simulink model "LinearSolver_System"  (R2021a)
settings: Solver=VariableStepAuto  StartTime=0.0  StopTime=1000  RelTol=1e-3
undefined symbols (not defined in the file or in its folder): AXI4, Lite
libraries: hdlBasic x415, xbsIndex_r4 x1
(part 1 of 4)
settings Model: Creator=hl116  LastModifiedBy=user

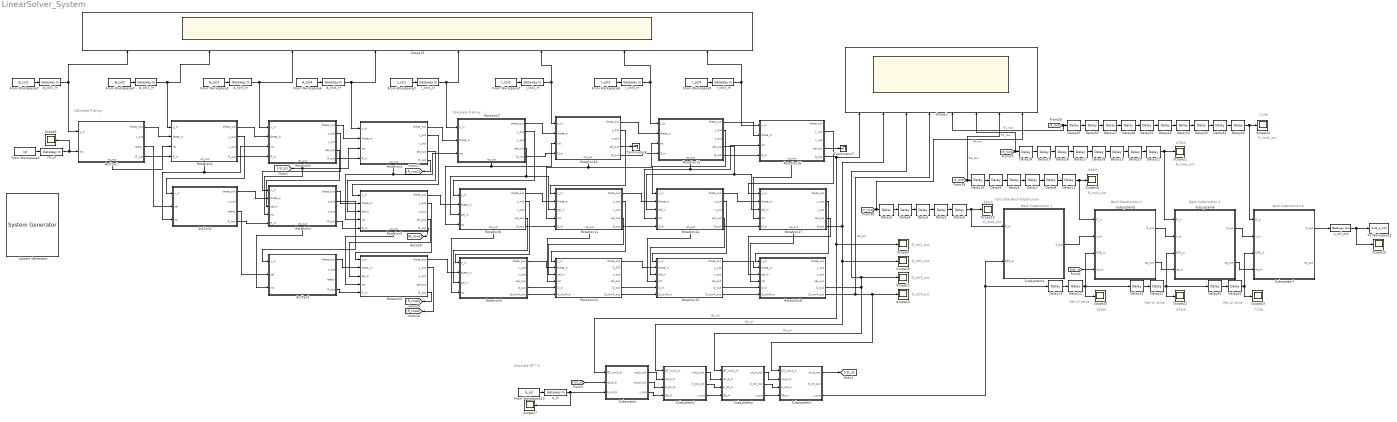
== system LinearSolver_System ==
  note: Q_col2_out
  note: 717th
  note: R_row1_out
  note: R_row3_out
  note: Q_col3_out
  note: Calculate QT * b
  note: 675th
  note: Calculate R Array
  note: y_out
  note: 717th
  note: Back Substitution 2
  note: Get y3 value
  note: Q_col1_out
  note: 633th
  note: 591th
  note: Calculate Q Array
  note: Back Substitution 4
  note: Back Substitution 1
  note: 675th
  note: Q_col4_out
  note: Get y2 value
  note: R_row2_out
  note: R_row4_out
  note: Get y2 value
  note: Calculate Back Substitution
  note: Back Substitution 3
  note: 633th
  " System Generator" : xbsIndex_r4/ System Generator  Tag=genX  xilinxfamily=zynq  part=xc7z020  speed=-1  package=clg484  synthesis_tool=Vivado  clock_wrapper=Clock Enables  directory=./netlist_project6_final  proj_type=Vivado  Synth_file=Vivado Synthesis Defaults  Impl_file=Vivado Implementation Defaults  testbench=off  simulink_period=1  sysclk_period=10  dcm_input_clock_period=10  incr_netlist=off  trim_vbits=Everywhere in SubSystem  dbl_ovrd=According to Block Masks  core_generation=According to Block Masks  run_coregen=off  deprecated_control=off  eval_field=0  block_type=sysgen
  A_col1_In : hdlBasic/Gateway In  gui_display_data_type=Fixed-point  arith_type=Signed (2's comp)  n_bits=16  bin_pt=13  preci_type=Single  exp_width=8  frac_width=24  rows=1  columns=1  quantization="Round  (unbiased: +/- Inf)"  overflow=Saturate  period=1  UseAsADC=off  ADCChannel='1'  interface=AXI4-Lite  automatic_assignment=on  address_offset=hex2dec('00')  intf_name=''  intf_description=''  default_value=0  timing_constraint=None  locs_specified=off  LOCs={}  io_standard={}  inherit_from_input=off  hdl_port=on  XmcBlockStatus=1  maskContainerNames=group4  block_type=gatewayin  block_config=sysgen:gateway_in_config  block_width_w=590  block_height_w=620  block_width=640  block_height=850
  A_col2_In : hdlBasic/Gateway In  gui_display_data_type=Fixed-point  arith_type=Signed (2's comp)  n_bits=16  bin_pt=13  preci_type=Single  exp_width=8  frac_width=24  rows=1  columns=1  quantization="Round  (unbiased: +/- Inf)"  overflow=Saturate  period=1  UseAsADC=off  ADCChannel='1'  interface=AXI4-Lite  automatic_assignment=on  address_offset=hex2dec('00')  intf_name=''  intf_description=''  default_value=0  timing_constraint=None  locs_specified=off  LOCs={}  io_standard={}  inherit_from_input=off  hdl_port=on  XmcBlockStatus=1  maskContainerNames=group4  block_type=gatewayin  block_config=sysgen:gateway_in_config  block_width_w=590  block_height_w=620  block_width=640  block_height=850
  A_col3_In : hdlBasic/Gateway In  gui_display_data_type=Fixed-point  arith_type=Signed (2's comp)  n_bits=16  bin_pt=13  preci_type=Single  exp_width=8  frac_width=24  rows=1  columns=1  quantization="Round  (unbiased: +/- Inf)"  overflow=Saturate  period=1  UseAsADC=off  ADCChannel='1'  interface=AXI4-Lite  automatic_assignment=on  address_offset=hex2dec('00')  intf_name=''  intf_description=''  default_value=0  timing_constraint=None  locs_specified=off  LOCs={}  io_standard={}  inherit_from_input=off  hdl_port=on  XmcBlockStatus=1  maskContainerNames=group4  block_type=gatewayin  block_config=sysgen:gateway_in_config  block_width_w=590  block_height_w=620  block_width=640  block_height=850
  A_col4_In : hdlBasic/Gateway In  gui_display_data_type=Fixed-point  arith_type=Signed (2's comp)  n_bits=16  bin_pt=13  preci_type=Single  exp_width=8  frac_width=24  rows=1  columns=1  quantization="Round  (unbiased: +/- Inf)"  overflow=Saturate  period=1  UseAsADC=off  ADCChannel='1'  interface=AXI4-Lite  automatic_assignment=on  address_offset=hex2dec('00')  intf_name=''  intf_description=''  default_value=0  timing_constraint=None  locs_specified=off  LOCs={}  io_standard={}  inherit_from_input=off  hdl_port=on  XmcBlockStatus=1  maskContainerNames=group4  block_type=gatewayin  block_config=sysgen:gateway_in_config  block_width_w=590  block_height_w=620  block_width=640  block_height=850
  ArcTan1 : Subsystem
      settings: PortSchema="{\"entries\":[{\"content\":{\"sides\":[{\"content\":{\"connectorIds\":[\"In1\",\"In2\"]},\"type\":\"ConnectorPlacement.EquallySpacedRectSide\",\"uuid\":\"caf108fa-2686-498d-a22a-9c5b9b2bbc42\"},{\"content\":{\"connectorIds\":[\"Out1\",\"Out2\",\"Out3\",\"Out4\"],\"side\":\"RIGHT\"},\"type\":\"ConnectorPlacement.EquallySpacedRectSide\",\"uuid\":\"907814ff-b94e-448a-ba79-154ff3b88489\"},{\"content\":{\"connectorIds\":[],\"side\":\"TOP\"},\"type\":\"ConnectorPlacement.EquallySpacedRectSide\",\"uuid\":\"95b6304b-e160-4f42-b0ad-ca1595d39137\"},{\"content\":{\"connectorIds\":[\"Out5\"],\"side\":\"BOTTOM\"},\"type\":\"ConnectorPlacement.EquallySpacedRectSide\",\"uuid\":\"89d2f461-a37a-483a-b43d-da0d10659910\"}]},\"type\":\"ConnectorPlacement.EquallySpacedConnector\",\"uuid\":\"3f5841f0-ef35-46d4-afb7-d5d76fae65b0\"}],\"packageUris\":[\"http://schema.mathworks.com/mf0/Connector/R2020b\"],\"version\":\"1.0\"}"
  ArcTan2 : Subsystem
  ArcTan3 : Subsystem
  Delay{1..35} (35 alike) : hdlBasic/Delay  rst=off  en=off  latency=42  reg_retiming=off  XmcBlockStatus=1  maskContainerNames=group1  block_type=delay  block_config=sysgen:Delay_config
  From Workspace1 : FromWorkspace  VariableName=I_col1
  From Workspace10 : FromWorkspace  VariableName=b_col
  From Workspace2 : FromWorkspace  VariableName=rst
  From Workspace3 : FromWorkspace  VariableName=A_col1
  From Workspace4 : FromWorkspace  VariableName=A_col2
  From Workspace5 : FromWorkspace  VariableName=A_col3
  From Workspace6 : FromWorkspace  VariableName=A_col4
  From Workspace7 : FromWorkspace  VariableName=I_col2
  From Workspace8 : FromWorkspace  VariableName=I_col3
  From Workspace9 : FromWorkspace  VariableName=I_col4
  I_col1_In : hdlBasic/Gateway In  gui_display_data_type=Fixed-point  arith_type=Signed (2's comp)  n_bits=16  bin_pt=13  preci_type=Single  exp_width=8  frac_width=24  rows=1  columns=1  quantization="Round  (unbiased: +/- Inf)"  overflow=Saturate  period=1  UseAsADC=off  ADCChannel='1'  interface=AXI4-Lite  automatic_assignment=on  address_offset=hex2dec('00')  intf_name=''  intf_description=''  default_value=0  timing_constraint=None  locs_specified=off  LOCs={}  io_standard={}  inherit_from_input=off  hdl_port=on  XmcBlockStatus=1  maskContainerNames=group4  block_type=gatewayin  block_config=sysgen:gateway_in_config  block_width_w=590  block_height_w=620  block_width=640  block_height=850
  I_col2_In : hdlBasic/Gateway In  gui_display_data_type=Fixed-point  arith_type=Signed (2's comp)  n_bits=16  bin_pt=13  preci_type=Single  exp_width=8  frac_width=24  rows=1  columns=1  quantization="Round  (unbiased: +/- Inf)"  overflow=Saturate  period=1  UseAsADC=off  ADCChannel='1'  interface=AXI4-Lite  automatic_assignment=on  address_offset=hex2dec('00')  intf_name=''  intf_description=''  default_value=0  timing_constraint=None  locs_specified=off  LOCs={}  io_standard={}  inherit_from_input=off  hdl_port=on  XmcBlockStatus=1  maskContainerNames=group4  block_type=gatewayin  block_config=sysgen:gateway_in_config  block_width_w=590  block_height_w=620  block_width=640  block_height=850
  I_col3_In : hdlBasic/Gateway In  gui_display_data_type=Fixed-point  arith_type=Signed (2's comp)  n_bits=16  bin_pt=13  preci_type=Single  exp_width=8  frac_width=24  rows=1  columns=1  quantization="Round  (unbiased: +/- Inf)"  overflow=Saturate  period=1  UseAsADC=off  ADCChannel='1'  interface=AXI4-Lite  automatic_assignment=on  address_offset=hex2dec('00')  intf_name=''  intf_description=''  default_value=0  timing_constraint=None  locs_specified=off  LOCs={}  io_standard={}  inherit_from_input=off  hdl_port=on  XmcBlockStatus=1  maskContainerNames=group4  block_type=gatewayin  block_config=sysgen:gateway_in_config  block_width_w=590  block_height_w=620  block_width=640  block_height=850
  I_col4_In : hdlBasic/Gateway In  gui_display_data_type=Fixed-point  arith_type=Signed (2's comp)  n_bits=16  bin_pt=13  preci_type=Single  exp_width=8  frac_width=24  rows=1  columns=1  quantization="Round  (unbiased: +/- Inf)"  overflow=Saturate  period=1  UseAsADC=off  ADCChannel='1'  interface=AXI4-Lite  automatic_assignment=on  address_offset=hex2dec('00')  intf_name=''  intf_description=''  default_value=0  timing_constraint=None  locs_specified=off  LOCs={}  io_standard={}  inherit_from_input=off  hdl_port=on  XmcBlockStatus=1  maskContainerNames=group4  block_type=gatewayin  block_config=sysgen:gateway_in_config  block_width_w=590  block_height_w=620  block_width=640  block_height=850
  Rotation1 : Subsystem
      settings: PortSchema="{\"entries\":[{\"content\":{\"sides\":[{\"content\":{\"connectorIds\":[\"In1\",\"In2\",\"In3\",\"In4\"]},\"type\":\"ConnectorPlacement.EquallySpacedRectSide\",\"uuid\":\"c3e45f34-1196-45a4-bcee-69f3d7240640\"},{\"content\":{\"connectorIds\":[\"Out1\",\"Out2\",\"Out3\",\"Out4\"],\"side\":\"RIGHT\"},\"type\":\"ConnectorPlacement.EquallySpacedRectSide\",\"uuid\":\"79e1b465-033e-4299-96e2-1b0cd35cf0c2\"},{\"content\":{\"connectorIds\":[],\"side\":\"TOP\"},\"type\":\"ConnectorPlacement.EquallySpacedRectSide\",\"uuid\":\"795b3f8d-3c8d-4387-9426-6b007387498d\"},{\"content\":{\"connectorIds\":[\"Out5\"],\"side\":\"BOTTOM\"},\"type\":\"ConnectorPlacement.EquallySpacedRectSide\",\"uuid\":\"45ba46a5-4748-4846-a91b-1f19bc6fdcdf\"}]},\"type\":\"ConnectorPlacement.EquallySpacedConnector\",\"uuid\":\"22f19e15-548a-4ba4-8f17-e0c3567ab6b5\"}],\"packageUris\":[\"http://schema.mathworks.com/mf0/Connector/R2020b\"],\"version\":\"1.0\"}"
  Rotation10 : Subsystem
      settings: PortSchema="{\"entries\":[{\"content\":{\"sides\":[{\"content\":{\"connectorIds\":[\"In1\",\"In2\",\"In3\",\"In4\"]},\"type\":\"ConnectorPlacement.EquallySpacedRectSide\",\"uuid\":\"068d33f8-cdb2-46c3-8301-e7e31b8e2d88\"},{\"content\":{\"connectorIds\":[\"Out1\",\"Out2\",\"Out3\",\"Out4\",\"Out5\"],\"side\":\"RIGHT\"},\"type\":\"ConnectorPlacement.EquallySpacedRectSide\",\"uuid\":\"83214df4-d8af-401f-bd94-7f29e76d3f14\"},{\"content\":{\"connectorIds\":[],\"side\":\"TOP\"},\"type\":\"ConnectorPlacement.EquallySpacedRectSide\",\"uuid\":\"05759f1c-0932-4c20-8c6f-a22efda59551\"},{\"content\":{\"connectorIds\":[\"Out6\"],\"side\":\"BOTTOM\"},\"type\":\"ConnectorPlacement.EquallySpacedRectSide\",\"uuid\":\"95c60bf2-d1b3-4d9f-8334-56ee824f5083\"}]},\"type\":\"ConnectorPlacement.EquallySpacedConnector\",\"uuid\":\"e196aaf4-fc67-40ce-aca9-a5a59584d6a1\"}],\"packageUris\":[\"http://schema.mathworks.com/mf0/Connector/R2020b\"],\"version\":\"1.0\"}"
  Rotation11 : Subsystem
      settings: PortSchema="{\"entries\":[{\"content\":{\"sides\":[{\"content\":{\"connectorIds\":[\"In1\",\"In2\",\"In3\",\"In4\",\"In5\"]},\"type\":\"ConnectorPlacement.EquallySpacedRectSide\",\"uuid\":\"6b6527a3-8e8e-46a8-ba4c-353728d938d4\"},{\"content\":{\"connectorIds\":[\"Out1\",\"Out2\",\"Out3\",\"Out4\",\"Out5\"],\"side\":\"RIGHT\"},\"type\":\"ConnectorPlacement.EquallySpacedRectSide\",\"uuid\":\"57a7f6f1-c89c-4a9c-80a9-96f08cfe423f\"},{\"content\":{\"connectorIds\":[],\"side\":\"TOP\"},\"type\":\"ConnectorPlacement.EquallySpacedRectSide\",\"uuid\":\"1e079b75-c7ea-4c6f-bb48-1f5f2befb45c\"},{\"content\":{\"connectorIds\":[\"Out6\"],\"side\":\"BOTTOM\"},\"type\":\"ConnectorPlacement.EquallySpacedRectSide\",\"uuid\":\"5c87db2d-8d39-4fe6-b9c8-0e27c9d7e4a1\"}]},\"type\":\"ConnectorPlacement.EquallySpacedConnector\",\"uuid\":\"501fe971-96c1-4a39-a71f-75caf46643d4\"}],\"packageUris\":[\"http://schema.mathworks.com/mf0/Connector/R2020b\"],\"version\":\"1.0\"}"
  Rotation12 : Subsystem
  Rotation13 : Subsystem
      settings: PortSchema="{\"entries\":[{\"content\":{\"sides\":[{\"content\":{\"connectorIds\":[\"In1\",\"In2\",\"In3\",\"In4\"]},\"type\":\"ConnectorPlacement.EquallySpacedRectSide\",\"uuid\":\"068d33f8-cdb2-46c3-8301-e7e31b8e2d88\"},{\"content\":{\"connectorIds\":[\"Out1\",\"Out2\",\"Out3\",\"Out4\",\"Out5\"],\"side\":\"RIGHT\"},\"type\":\"ConnectorPlacement.EquallySpacedRectSide\",\"uuid\":\"83214df4-d8af-401f-bd94-7f29e76d3f14\"},{\"content\":{\"connectorIds\":[],\"side\":\"TOP\"},\"type\":\"ConnectorPlacement.EquallySpacedRectSide\",\"uuid\":\"05759f1c-0932-4c20-8c6f-a22efda59551\"},{\"content\":{\"connectorIds\":[\"Out6\"],\"side\":\"BOTTOM\"},\"type\":\"ConnectorPlacement.EquallySpacedRectSide\",\"uuid\":\"4a007575-1088-4b4a-8c4b-3cebef37980c\"}]},\"type\":\"ConnectorPlacement.EquallySpacedConnector\",\"uuid\":\"e196aaf4-fc67-40ce-aca9-a5a59584d6a1\"}],\"packageUris\":[\"http://schema.mathworks.com/mf0/Connector/R2020b\"],\"version\":\"1.0\"}"
  Rotation14 : Subsystem
      settings: PortSchema="{\"entries\":[{\"content\":{\"sides\":[{\"content\":{\"connectorIds\":[\"In1\",\"In2\",\"In3\",\"In4\",\"In5\"]},\"type\":\"ConnectorPlacement.EquallySpacedRectSide\",\"uuid\":\"6b6527a3-8e8e-46a8-ba4c-353728d938d4\"},{\"content\":{\"connectorIds\":[\"Out1\",\"Out2\",\"Out3\",\"Out4\",\"Out5\"],\"side\":\"RIGHT\"},\"type\":\"ConnectorPlacement.EquallySpacedRectSide\",\"uuid\":\"57a7f6f1-c89c-4a9c-80a9-96f08cfe423f\"},{\"content\":{\"connectorIds\":[],\"side\":\"TOP\"},\"type\":\"ConnectorPlacement.EquallySpacedRectSide\",\"uuid\":\"1e079b75-c7ea-4c6f-bb48-1f5f2befb45c\"},{\"content\":{\"connectorIds\":[\"Out6\"],\"side\":\"BOTTOM\"},\"type\":\"ConnectorPlacement.EquallySpacedRectSide\",\"uuid\":\"061fd00d-29db-46d9-9c72-ed1c1f9fbab0\"}]},\"type\":\"ConnectorPlacement.EquallySpacedConnector\",\"uuid\":\"501fe971-96c1-4a39-a71f-75caf46643d4\"}],\"packageUris\":[\"http://schema.mathworks.com/mf0/Connector/R2020b\"],\"version\":\"1.0\"}"
  Rotation15 : Subsystem
  Rotation16 : Subsystem
      settings: PortSchema="{\"entries\":[{\"content\":{\"sides\":[{\"content\":{\"connectorIds\":[\"In1\",\"In2\",\"In3\",\"In4\"]},\"type\":\"ConnectorPlacement.EquallySpacedRectSide\",\"uuid\":\"068d33f8-cdb2-46c3-8301-e7e31b8e2d88\"},{\"content\":{\"connectorIds\":[\"Out1\",\"Out2\",\"Out3\",\"Out4\",\"Out5\"],\"side\":\"RIGHT\"},\"type\":\"ConnectorPlacement.EquallySpacedRectSide\",\"uuid\":\"83214df4-d8af-401f-bd94-7f29e76d3f14\"},{\"content\":{\"connectorIds\":[],\"side\":\"TOP\"},\"type\":\"ConnectorPlacement.EquallySpacedRectSide\",\"uuid\":\"05759f1c-0932-4c20-8c6f-a22efda59551\"},{\"content\":{\"connectorIds\":[\"Out6\"],\"side\":\"BOTTOM\"},\"type\":\"ConnectorPlacement.EquallySpacedRectSide\",\"uuid\":\"a5d5f222-4f9a-4dec-95b1-9bb538967935\"}]},\"type\":\"ConnectorPlacement.EquallySpacedConnector\",\"uuid\":\"e196aaf4-fc67-40ce-aca9-a5a59584d6a1\"}],\"packageUris\":[\"http://schema.mathworks.com/mf0/Connector/R2020b\"],\"version\":\"1.0\"}"
  Rotation17 : Subsystem
      settings: PortSchema="{\"entries\":[{\"content\":{\"sides\":[{\"content\":{\"connectorIds\":[\"In1\",\"In2\",\"In3\",\"In4\",\"In5\"]},\"type\":\"ConnectorPlacement.EquallySpacedRectSide\",\"uuid\":\"6b6527a3-8e8e-46a8-ba4c-353728d938d4\"},{\"content\":{\"connectorIds\":[\"Out1\",\"Out2\",\"Out3\",\"Out4\",\"Out5\"],\"side\":\"RIGHT\"},\"type\":\"ConnectorPlacement.EquallySpacedRectSide\",\"uuid\":\"57a7f6f1-c89c-4a9c-80a9-96f08cfe423f\"},{\"content\":{\"connectorIds\":[],\"side\":\"TOP\"},\"type\":\"ConnectorPlacement.EquallySpacedRectSide\",\"uuid\":\"1e079b75-c7ea-4c6f-bb48-1f5f2befb45c\"},{\"content\":{\"connectorIds\":[\"Out6\"],\"side\":\"BOTTOM\"},\"type\":\"ConnectorPlacement.EquallySpacedRectSide\",\"uuid\":\"3587cf55-3b2f-4d34-81c4-8d2cc648f644\"}]},\"type\":\"ConnectorPlacement.EquallySpacedConnector\",\"uuid\":\"501fe971-96c1-4a39-a71f-75caf46643d4\"}],\"packageUris\":[\"http://schema.mathworks.com/mf0/Connector/R2020b\"],\"version\":\"1.0\"}"
  Rotation18 : Subsystem
  Rotation2 : Subsystem
      settings: PortSchema="{\"entries\":[{\"content\":{\"sides\":[{\"content\":{\"connectorIds\":[\"In1\",\"In2\",\"In3\",\"In4\"]},\"type\":\"ConnectorPlacement.EquallySpacedRectSide\",\"uuid\":\"068d33f8-cdb2-46c3-8301-e7e31b8e2d88\"},{\"content\":{\"connectorIds\":[\"Out1\",\"Out2\",\"Out3\",\"Out4\",\"Out5\"],\"side\":\"RIGHT\"},\"type\":\"ConnectorPlacement.EquallySpacedRectSide\",\"uuid\":\"83214df4-d8af-401f-bd94-7f29e76d3f14\"},{\"content\":{\"connectorIds\":[],\"side\":\"TOP\"},\"type\":\"ConnectorPlacement.EquallySpacedRectSide\",\"uuid\":\"05759f1c-0932-4c20-8c6f-a22efda59551\"},{\"content\":{\"connectorIds\":[\"Out6\"],\"side\":\"BOTTOM\"},\"type\":\"ConnectorPlacement.EquallySpacedRectSide\",\"uuid\":\"987827c9-e6f7-4c94-aabc-7251ec600981\"}]},\"type\":\"ConnectorPlacement.EquallySpacedConnector\",\"uuid\":\"e196aaf4-fc67-40ce-aca9-a5a59584d6a1\"}],\"packageUris\":[\"http://schema.mathworks.com/mf0/Connector/R2020b\"],\"version\":\"1.0\"}"
  Rotation3 : Subsystem
      settings: PortSchema="{\"entries\":[{\"content\":{\"sides\":[{\"content\":{\"connectorIds\":[\"In1\",\"In2\",\"In3\",\"In4\",\"In5\"]},\"type\":\"ConnectorPlacement.EquallySpacedRectSide\",\"uuid\":\"5a2488f2-5ccf-45a0-803f-ac02516baf2a\"},{\"content\":{\"connectorIds\":[\"Out1\",\"Out2\",\"Out3\",\"Out4\"],\"side\":\"RIGHT\"},\"type\":\"ConnectorPlacement.EquallySpacedRectSide\",\"uuid\":\"04a338b1-3409-43d4-bd2c-1e3a68bdc033\"},{\"content\":{\"connectorIds\":[],\"side\":\"TOP\"},\"type\":\"ConnectorPlacement.EquallySpacedRectSide\",\"uuid\":\"c32ba394-10a6-4b90-81f2-7c803e47e1d6\"},{\"content\":{\"connectorIds\":[\"Out5\"],\"side\":\"BOTTOM\"},\"type\":\"ConnectorPlacement.EquallySpacedRectSide\",\"uuid\":\"b18b14a5-9051-48c4-88ed-3c7a3a432492\"}]},\"type\":\"ConnectorPlacement.EquallySpacedConnector\",\"uuid\":\"22fd47f4-abd7-42f1-b7d4-b847dde25346\"}],\"packageUris\":[\"http://schema.mathworks.com/mf0/Connector/R2020b\"],\"version\":\"1.0\"}"
  Rotation4 : Subsystem
      settings: PortSchema="{\"entries\":[{\"content\":{\"sides\":[{\"content\":{\"connectorIds\":[\"In1\",\"In2\",\"In3\",\"In4\"]},\"type\":\"ConnectorPlacement.EquallySpacedRectSide\",\"uuid\":\"068d33f8-cdb2-46c3-8301-e7e31b8e2d88\"},{\"content\":{\"connectorIds\":[\"Out1\",\"Out2\",\"Out3\",\"Out4\",\"Out5\"],\"side\":\"RIGHT\"},\"type\":\"ConnectorPlacement.EquallySpacedRectSide\",\"uuid\":\"83214df4-d8af-401f-bd94-7f29e76d3f14\"},{\"content\":{\"connectorIds\":[],\"side\":\"TOP\"},\"type\":\"ConnectorPlacement.EquallySpacedRectSide\",\"uuid\":\"05759f1c-0932-4c20-8c6f-a22efda59551\"},{\"content\":{\"connectorIds\":[\"Out6\"],\"side\":\"BOTTOM\"},\"type\":\"ConnectorPlacement.EquallySpacedRectSide\",\"uuid\":\"07663304-5c03-41b4-8589-fbaa6acb83e6\"}]},\"type\":\"ConnectorPlacement.EquallySpacedConnector\",\"uuid\":\"e196aaf4-fc67-40ce-aca9-a5a59584d6a1\"}],\"packageUris\":[\"http://schema.mathworks.com/mf0/Connector/R2020b\"],\"version\":\"1.0\"}"
  Rotation5 : Subsystem
      settings: PortSchema="{\"entries\":[{\"content\":{\"sides\":[{\"content\":{\"connectorIds\":[\"In1\",\"In2\",\"In3\",\"In4\",\"In5\"]},\"type\":\"ConnectorPlacement.EquallySpacedRectSide\",\"uuid\":\"6b6527a3-8e8e-46a8-ba4c-353728d938d4\"},{\"content\":{\"connectorIds\":[\"Out1\",\"Out2\",\"Out3\",\"Out4\",\"Out5\"],\"side\":\"RIGHT\"},\"type\":\"ConnectorPlacement.EquallySpacedRectSide\",\"uuid\":\"57a7f6f1-c89c-4a9c-80a9-96f08cfe423f\"},{\"content\":{\"connectorIds\":[],\"side\":\"TOP\"},\"type\":\"ConnectorPlacement.EquallySpacedRectSide\",\"uuid\":\"1e079b75-c7ea-4c6f-bb48-1f5f2befb45c\"},{\"content\":{\"connectorIds\":[\"Out6\"],\"side\":\"BOTTOM\"},\"type\":\"ConnectorPlacement.EquallySpacedRectSide\",\"uuid\":\"f0f6f5df-f68e-427f-a9b7-f2b0f67ab02e\"}]},\"type\":\"ConnectorPlacement.EquallySpacedConnector\",\"uuid\":\"501fe971-96c1-4a39-a71f-75caf46643d4\"}],\"packageUris\":[\"http://schema.mathworks.com/mf0/Connector/R2020b\"],\"version\":\"1.0\"}"
  Rotation6 : Subsystem
  Rotation7 : Subsystem
      settings: PortSchema="{\"entries\":[{\"content\":{\"sides\":[{\"content\":{\"connectorIds\":[\"In1\",\"In2\",\"In3\"]},\"type\":\"ConnectorPlacement.EquallySpacedRectSide\",\"uuid\":\"1e76d85c-3914-4810-b88f-69e12f1ce3e7\"},{\"content\":{\"connectorIds\":[\"Out1\",\"Out2\",\"Out3\",\"Out4\",\"Out5\"],\"side\":\"RIGHT\"},\"type\":\"ConnectorPlacement.EquallySpacedRectSide\",\"uuid\":\"b2a3ae44-27c5-4e6a-a77b-0f976930a7b4\"},{\"content\":{\"connectorIds\":[],\"side\":\"TOP\"},\"type\":\"ConnectorPlacement.EquallySpacedRectSide\",\"uuid\":\"79a2ca68-cad6-41af-8f6d-116779ed3f68\"},{\"content\":{\"connectorIds\":[\"Out6\"],\"side\":\"BOTTOM\"},\"type\":\"ConnectorPlacement.EquallySpacedRectSide\",\"uuid\":\"00f5f418-aace-4f23-81ae-265cee9e2cf4\"}]},\"type\":\"ConnectorPlacement.EquallySpacedConnector\",\"uuid\":\"569dc780-af12-452d-86d9-ad002fe759ae\"}],\"packageUris\":[\"http://schema.mathworks.com/mf0/Connector/R2020b\"],\"version\":\"1.0\"}"
  Rotation8 : Subsystem
      settings: PortSchema="{\"entries\":[{\"content\":{\"sides\":[{\"content\":{\"connectorIds\":[\"In1\",\"In2\",\"In3\",\"In4\"]},\"type\":\"ConnectorPlacement.EquallySpacedRectSide\",\"uuid\":\"068d33f8-cdb2-46c3-8301-e7e31b8e2d88\"},{\"content\":{\"connectorIds\":[\"Out1\",\"Out2\",\"Out3\",\"Out4\",\"Out5\"],\"side\":\"RIGHT\"},\"type\":\"ConnectorPlacement.EquallySpacedRectSide\",\"uuid\":\"83214df4-d8af-401f-bd94-7f29e76d3f14\"},{\"content\":{\"connectorIds\":[],\"side\":\"TOP\"},\"type\":\"ConnectorPlacement.EquallySpacedRectSide\",\"uuid\":\"05759f1c-0932-4c20-8c6f-a22efda59551\"},{\"content\":{\"connectorIds\":[\"Out6\"],\"side\":\"BOTTOM\"},\"type\":\"ConnectorPlacement.EquallySpacedRectSide\",\"uuid\":\"ce8defe0-48f5-4c2d-b931-15403bf1b1bf\"}]},\"type\":\"ConnectorPlacement.EquallySpacedConnector\",\"uuid\":\"e196aaf4-fc67-40ce-aca9-a5a59584d6a1\"}],\"packageUris\":[\"http://schema.mathworks.com/mf0/Connector/R2020b\"],\"version\":\"1.0\"}"
  Rotation9 : Subsystem
  Scope1 : Scope  NumInputPorts=8
  Scope{2,9..12,17..25} (14 alike) : Scope
  Scope13 : Scope  NumInputPorts=8
  Subsystem : Subsystem
  Subsystem1 : Subsystem
  Subsystem2 : Subsystem
  Subsystem3 : Subsystem
  Subsystem4 : Subsystem
  Subsystem5 : Subsystem
  Subsystem6 : Subsystem
  Subsystem7 : Subsystem
  Terminator4 : Terminator
  Terminator7 : Terminator
  To Workspace1 : ToWorkspace  VariableName=out_x_col  SampleTime=-1
  b_In : hdlBasic/Gateway In  gui_display_data_type=Fixed-point  arith_type=Signed (2's comp)  n_bits=16  bin_pt=13  preci_type=Single  exp_width=8  frac_width=24  rows=1  columns=1  quantization="Round  (unbiased: +/- Inf)"  overflow=Saturate  period=1  UseAsADC=off  ADCChannel='1'  interface=AXI4-Lite  automatic_assignment=on  address_offset=hex2dec('00')  intf_name=''  intf_description=''  default_value=0  timing_constraint=None  locs_specified=off  LOCs={}  io_standard={}  inherit_from_input=off  hdl_port=on  XmcBlockStatus=1  maskContainerNames=group4  block_type=gatewayin  block_config=sysgen:gateway_in_config  block_width_w=590  block_height_w=620  block_width=640  block_height=850
  rst_In : hdlBasic/Gateway In  gui_display_data_type=Boolean  arith_type=Boolean  n_bits=16  bin_pt=13  preci_type=Single  exp_width=8  frac_width=24  rows=1  columns=1  quantization="Round  (unbiased: +/- Inf)"  overflow=Saturate  period=1  UseAsADC=off  ADCChannel='1'  interface=AXI4-Lite  automatic_assignment=on  address_offset=hex2dec('00')  intf_name=''  intf_description=''  default_value=0  timing_constraint=None  locs_specified=off  LOCs={}  io_standard={}  inherit_from_input=off  hdl_port=on  XmcBlockStatus=1  maskContainerNames=group4  block_type=gatewayin  block_config=sysgen:gateway_in_config  block_width_w=590  block_height_w=620  block_width=640  block_height=850
  x_col_out : hdlBasic/Gateway Out  inherit_from_input=off  hdl_port=on  rows=1  columns=1  UseAsDAC=off  DACChannel='1'  interface=AXI4-Lite  automatic_assignment=on  address_offset=hex2dec('00')  intf_name=''  intf_description=''  timing_constraint=None  locs_specified=off  LOCs={}  io_standard={}  XmcBlockStatus=1  maskContainerNames=group4  block_type=gatewayout  block_config=sysgen:gateway_out_config  block_width_w=590  block_height_w=620  block_width=620  block_height=750
  wires:
  x_col_out/1 -> Scope25/1, To Workspace1/1
  Delay32/1 -> Delay33/1
  Subsystem1/2(b_col_out) -> Subsystem2/3(b_col_In)
  ArcTan2/4(R_out) -> Rotation3/5(R_in)
  Rotation5/5(R_out) -> [R_row2]
  Rotation14/1(theta_out) -> Rotation17/2(theta_in)
  Delay35/1 -> Delay24/1
  From Workspace1/1 -> I_col1_In/1
  Delay15/1 -> Delay20/1
  Rotation4/5(R_out) -> [R_row1]
  Rotation2/5(R_out) -> Rotation4/4(R_in)
  Delay19/1 -> Delay16/1
  Delay6/1 -> Delay7/1
  Rotation3/1(theta_out) -> Rotation5/2(theta_in)
  Delay33/1 -> Delay34/1
  Subsystem/2(b_col_out) -> Subsystem1/3(b_col_In)
  Delay34/1 -> Subsystem7/1(R_in), Scope24/1
  Delay1/1 -> Delay2/1
  Rotation7/5(Q_out) -> Rotation10/4(Q_in)
  Rotation13/4(sel_out) -> Rotation17/3(sel_in), Rotation14/3(sel_in)
  [rst_b] -> Subsystem/2(rst_b_In)
  Rotation7/2(y_out) -> Rotation8/1(y_in)
  Rotation11/5(Q_out) -> Rotation14/5(Q_in)
  Subsystem/3(y_out) -> Subsystem1/4(Qb_In)
  From Workspace10/1 -> b_In/1
  Rotation1/5(rst_out) -> ArcTan2/3(rst), Rotation2/3(rst)
  I_col1_In/1 -> Scope13/5, Rotation7/1(y_in)
  A_col1_In/1 -> Scope13/1, ArcTan1/1(y_in)
  b_In/1 -> Scope17/1, Subsystem/3(b_col_In)
  Rotation12/6(Q_row4_out) -> Rotation15/6(Q_row4_in)
  Rotation6/1(theta_out) -> Rotation9/2(theta_in)
  A_col2_In/1 -> Scope13/2, Rotation1/1(y_in)
  Rotation9/6(Q_row4_out) -> Rotation12/6(Q_row4_in)
  Rotation8/1(theta_out) -> Rotation11/2(theta_in)
  Rotation7/6(rst_out) -> Rotation8/4(rst), Rotation10/3(rst)
  Rotation15/1(theta_out) -> Rotation18/2(theta_in)
  Rotation10/2(y_out) -> Rotation11/1(y_in)
  ArcTan1/1(theta_out) -> Rotation1/2(theta_in)
  Rotation14/2(y_out) -> Rotation15/1(y_in)
  Rotation16/5(Q_out) -> Scope1/1, Scope9/1, Subsystem/1(QT_row1_In)  "Q1_col"
  Rotation2/4(sel_out) -> Rotation3/3(sel_in)
  Rotation4/6(rst_out) -> Rotation7/3(rst), Rotation5/4(rst)
  ArcTan1/3(ready) -> ArcTan2/2(sel)
  Rotation1/4(R_out) -> Rotation2/4(R_in)
  Rotation8/5(Q_out) -> Rotation11/5(Q_in)
  From Workspace2/1 -> rst_In/1
  Rotation6/2(y_out) -> [R_row4]
  Rotation11/4(sel_out) -> Rotation12/3(sel_in)
  Rotation17/2(y_out) -> Rotation18/1(y_in)
  Rotation1/1(theta_out) -> Rotation2/2(theta_in)
  A_col3_In/1 -> Scope13/3, Rotation2/1(y_in)
  [R_row4] -> Delay5/1, Scope1/8  "R4_row"
  rst_In/1 -> Scope2/1, ArcTan1/2(rst)
  Rotation9/1(theta_out) -> Rotation12/2(theta_in)
  A_col4_In/1 -> Scope13/4, Rotation4/1(y_in)
  Rotation11/2(y_out) -> Rotation12/1(y_in)
  Rotation13/1(theta_out) -> Rotation16/2(theta_in)
  Rotation6/5(R_out) -> [R_row3]
  Rotation10/5(Q_out) -> Rotation13/4(Q_in)
  Rotation14/6(rst_out) -> Rotation15/4(rst)
  Rotation12/1(theta_out) -> Rotation15/2(theta_in)
  Delay31/1 -> Delay32/1
  ArcTan1/5(rst_out) -> Rotation1/3(rst)
  Rotation2/1(theta_out) -> Rotation4/2(theta_in)
  Rotation2/6(rst_out) -> Rotation3/4(rst), Rotation4/3(rst), [rst_b]
  Rotation11/6(rst_out) -> Rotation12/4(rst)
  I_col4_In/1 -> Scope13/8, Rotation16/1(y_in)
  Subsystem7/1(X_out) -> x_col_out/1
  From Workspace6/1 -> A_col4_In/1
  [R_row2] -> Scope1/6, Delay14/1  "R2_row"
  Rotation2/2(y_out) -> Rotation3/1(y_in)
  [R_row1] -> Delay25/1, Scope1/5  "R1_row"
  Rotation15/5(Q_out) -> Rotation18/5(Q_in)
  Rotation17/6(rst_out) -> Rotation18/4(rst)
  Rotation5/4(sel_out) -> Rotation6/3(sel_in)
  Rotation18/5(Q_out) -> Scope11/1, Scope1/3, Subsystem2/1(QT_row3_In)  "Q3_col"
  From Workspace4/1 -> A_col2_In/1
  Rotation1/2(y_out) -> ArcTan2/1(y_in)
  From Workspace5/1 -> A_col3_In/1
  Rotation4/2(y_out) -> Rotation5/1(y_in)
  Delay17/1 -> Delay18/1
  Rotation8/4(sel_out) -> Rotation9/3(sel_in)
  Subsystem5/2(rst_out) -> Subsystem6/4(rst_in)
  Rotation3/2(y_out) -> ArcTan3/1(y_in)
  Delay18/1 -> Delay15/1
  Subsystem6/2(rst_out) -> Subsystem7/4(rst_in)
  Rotation10/4(sel_out) -> Terminator4/1
  Delay26/1 -> Delay31/1
  Delay3/1 -> Subsystem4/1(R_in), Scope19/1
  Rotation15/6(Q_row4_out) -> Rotation18/6(Q_row4_in)
  Rotation8/6(rst_out) -> Rotation9/4(rst)
  From Workspace3/1 -> A_col1_In/1
  Delay28/1 -> Delay29/1
  Rotation9/5(Q_out) -> Rotation12/5(Q_in)
  Delay25/1 -> Delay30/1
  Delay30/1 -> Delay27/1
  Rotation5/2(y_out) -> Rotation6/1(y_in)
  Delay24/1 -> Subsystem7/3(QTb_in), Scope23/1
  Rotation12/5(Q_out) -> Rotation15/5(Q_in)
  Delay27/1 -> Delay28/1
  From Workspace9/1 -> I_col4_In/1
  Rotation13/5(Q_out) -> Rotation16/4(Q_in)
  Delay22/1 -> Delay35/1, Subsystem6/3(QTb_in), Scope22/1
  Subsystem6/1(X_out) -> Subsystem7/2(x_in)
  ArcTan2/3(ready) -> ArcTan3/2(sel)
  ArcTan1/4(R_out) -> Rotation1/4(R_in)
  [rst_x] -> Subsystem5/4(rst_in)
  Rotation4/1(theta_out) -> Rotation7/2(theta_in)
  Rotation13/2(y_out) -> Rotation14/1(y_in)
  Rotation10/1(theta_out) -> Rotation13/2(theta_in)
  Delay23/1 -> Delay22/1
  I_col2_In/1 -> Scope13/6, Rotation10/1(y_in)
  Rotation3/5(rst_out) -> ArcTan3/3(rst)
  Delay5/1 -> Delay4/1
  Rotation5/1(theta_out) -> Rotation8/2(theta_in)
  Rotation7/1(theta_out) -> Rotation10/2(theta_in)
  Rotation11/1(theta_out) -> Rotation14/2(theta_in)
  Subsystem3/1(rst_b_out) -> [rst_x]
  I_col3_In/1 -> Scope13/7, Rotation13/1(y_in)
  Delay14/1 -> Delay19/1
  Subsystem4/1(X_out) -> Subsystem5/2(x_in)
  Delay12/1 -> Scope20/1, Delay23/1, Subsystem5/3(QTb_in)
  [R_row3] -> Scope1/7, Delay10/1  "R3_row"
  Delay8/1 -> Delay11/1
  ArcTan2/1(theta_out) -> Rotation3/2(theta_in)
  Delay9/1 -> Delay6/1
  Delay13/1 -> Delay12/1
  Rotation17/4(sel_out) -> Rotation18/3(sel_in)
  Rotation4/4(sel_out) -> Rotation5/3(sel_in)
  From Workspace8/1 -> I_col3_In/1
  Subsystem5/1(X_out) -> Subsystem6/2(x_in)
  From Workspace7/1 -> I_col2_In/1
  Delay7/1 -> Delay8/1
  Rotation13/6(rst_out) -> Rotation14/4(rst), Rotation16/3(rst)
  Delay10/1 -> Delay9/1
  Rotation18/6(Q_row4_out) -> Scope12/1, Subsystem3/1(QT_row4_In), Scope1/4  "Q4_col"
  ArcTan3/1(theta_out) -> Rotation6/2(theta_in)
  Subsystem3/3(y_out) -> Delay13/1, Subsystem4/2(QTb_in)
  Rotation7/4(sel_out) -> Rotation11/3(sel_in), Rotation8/3(sel_in)
  ArcTan3/4(R_out) -> Rotation6/5(R_in)
  Rotation16/2(y_out) -> Rotation17/1(y_in)
  Subsystem1/1(rst_b_out) -> Subsystem2/2(rst_b_In)
  Rotation3/4(R_out) -> Rotation5/5(R_in)
  Delay20/1 -> Delay21/1
  Rotation10/6(rst_out) -> Rotation11/4(rst), Rotation13/3(rst)
  Delay2/1 -> Delay3/1
  Delay11/1 -> Scope18/1, Subsystem5/1(R_in)
  Subsystem/1(rst_b_out) -> Subsystem1/2(rst_b_In)
  Delay16/1 -> Delay17/1
  Rotation17/5(Q_out) -> Scope10/1, Subsystem1/1(QT_row2_In), Scope1/2  "Q2_col"
  Rotation14/4(sel_out) -> Rotation15/3(sel_in)
  Subsystem2/1(rst_b_out) -> Subsystem3/2(rst_b_In)
  Rotation5/6(rst_out) -> Rotation6/4(rst)
  Delay29/1 -> Delay26/1
  Rotation16/6(rst_out) -> Rotation17/4(rst)
  Delay4/1 -> Delay1/1
  Subsystem2/2(b_col_out) -> Subsystem3/3(b_col_In)
  Subsystem1/3(y_out) -> Subsystem2/4(Qb_In)
  Rotation16/4(sel_out) -> Terminator7/1
  Subsystem2/3(y_out) -> Subsystem3/4(Qb_In)
  Rotation8/2(y_out) -> Rotation9/1(y_in)
  Delay21/1 -> Subsystem6/1(R_in), Scope21/1
  Rotation14/5(Q_out) -> Rotation17/5(Q_in)

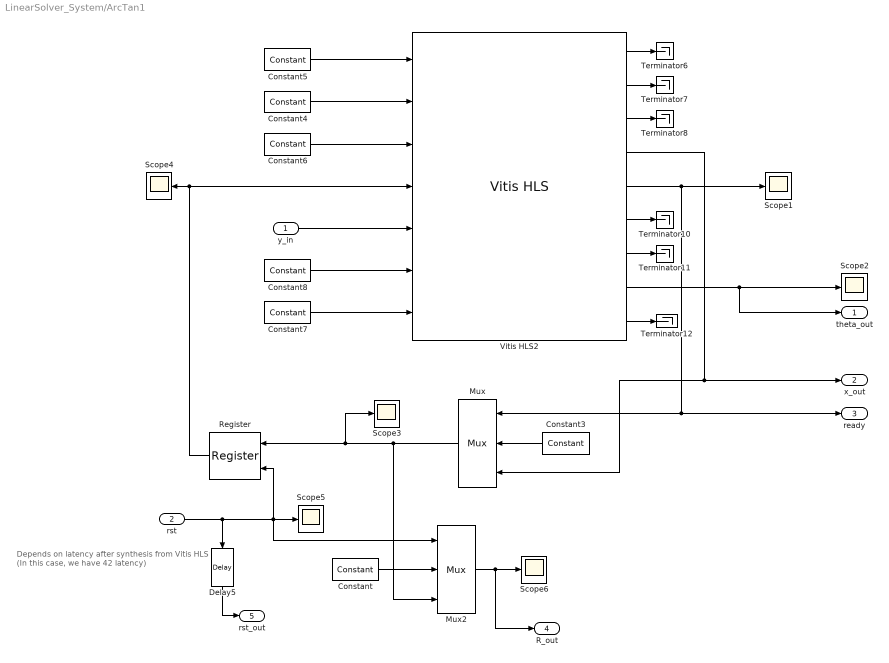
== system LinearSolver_System/ArcTan1 ==
  note: Depends on latency
      | after synthesis from Vitis HLS
      | (In this case, we have 42 latency)
  y_in : Inport
  rst : Inport  Port=2
  Constant : hdlBasic/Constant  const=0  gui_display_data_type=Fixed-point  arith_type=Signed (2's comp)  n_bits=16  bin_pt=13  preci_type=Single  exp_width=8  frac_width=24  explicit_period=off  period=1  XmcBlockStatus=1  maskContainerNames=tabcontainer1  block_type=constant  block_config=sysgen:Constant_config
  Constant3 : hdlBasic/Constant  const=0.0  gui_display_data_type=Fixed-point  arith_type=Signed (2's comp)  n_bits=16  bin_pt=13  preci_type=Single  exp_width=8  frac_width=24  explicit_period=off  period=1  XmcBlockStatus=1  maskContainerNames=tabcontainer1  block_type=constant  block_config=sysgen:Constant_config
  Constant4 : hdlBasic/Constant  const=1.0  gui_display_data_type=Boolean  arith_type=Boolean  n_bits=16  bin_pt=14  preci_type=Single  exp_width=8  frac_width=24  explicit_period=off  period=1  XmcBlockStatus=1  maskContainerNames=tabcontainer1  block_type=constant  block_config=sysgen:Constant_config
  Constant5 : hdlBasic/Constant  const=0  gui_display_data_type=Boolean  arith_type=Boolean  n_bits=16  bin_pt=14  preci_type=Single  exp_width=8  frac_width=24  explicit_period=off  period=1  XmcBlockStatus=1  maskContainerNames=tabcontainer1  block_type=constant  block_config=sysgen:Constant_config
  Constant6 : hdlBasic/Constant  const=1  gui_display_data_type=Boolean  arith_type=Boolean  n_bits=16  bin_pt=13  preci_type=Single  exp_width=8  frac_width=24  explicit_period=off  period=1  XmcBlockStatus=1  maskContainerNames=tabcontainer1  block_type=constant  block_config=sysgen:Constant_config
  Constant7 : hdlBasic/Constant  const=0.0  gui_display_data_type=Fixed-point  arith_type=Signed (2's comp)  n_bits=16  bin_pt=0  preci_type=Single  exp_width=8  frac_width=24  explicit_period=off  period=1  XmcBlockStatus=1  maskContainerNames=tabcontainer1  block_type=constant  block_config=sysgen:Constant_config
  Constant8 : hdlBasic/Constant  const=0.0  gui_display_data_type=Fixed-point  arith_type=Signed (2's comp)  n_bits=16  bin_pt=13  preci_type=Single  exp_width=8  frac_width=24  explicit_period=off  period=1  XmcBlockStatus=1  maskContainerNames=tabcontainer1  block_type=constant  block_config=sysgen:Constant_config
  Delay5 : hdlBasic/Delay  rst=off  en=off  latency=42  reg_retiming=off  XmcBlockStatus=1  maskContainerNames=group1  block_type=delay  block_config=sysgen:Delay_config
  Mux : hdlBasic/Mux  inputs=2  en=off  latency=0  precision=Full  arith_type=Unsigned  n_bits=16  bin_pt=14  quantization=Truncate  overflow=Wrap  XmcBlockStatus=1  maskContainerNames=tabcontainer1  block_type=mux  block_config=sysgen:Mux_config
  Mux2 : hdlBasic/Mux  inputs=2  en=off  latency=0  precision=Full  arith_type=Unsigned  n_bits=16  bin_pt=14  quantization=Truncate  overflow=Wrap  XmcBlockStatus=1  maskContainerNames=tabcontainer1  block_type=mux  block_config=sysgen:Mux_config
  Register : hdlBasic/Register  init=0  rst=on  en=off  XmcBlockStatus=1  maskContainerNames=tabcontainer1  block_type=register  block_config=sysgen:Register_config
  Scope{1..6} (6 alike) : Scope
  Terminator{6..8,10..12} (6 alike) : Terminator
  Vitis HLS2 : hdlBasic/Vitis HLS  anytable='..\Vitis_HLS\project6_final_hls_mc\solution1_without_back_substitution'  fast_sim=off  display_datatype=off  rate_propagation_method=Simulink system period  model_file_path=''  latency=1  block_type=vitis_hls
      settings: infoedit=This block allows including C,C++ and SystemC source files in System Generator for DSP designs.
  theta_out : Outport
  x_out : Outport  Port=2
  ready : Outport  Port=3
  R_out : Outport  Port=4
  rst_out : Outport  Port=5
  wires:
  Constant3/1 -> Mux/2
  Mux/1 -> Scope3/1, Register/1, Mux2/3
  y_in/1 -> Vitis HLS2/5
  Register/1 -> Scope4/1, Vitis HLS2/4
  Vitis HLS2/4 -> x_out/1, Mux/3
  Vitis HLS2/5 -> Scope1/1, ready/1, Mux/1
  Constant5/1 -> Vitis HLS2/1
  Constant4/1 -> Vitis HLS2/2
  Constant6/1 -> Vitis HLS2/3
  Vitis HLS2/1 -> Terminator6/1
  Vitis HLS2/2 -> Terminator7/1
  Vitis HLS2/3 -> Terminator8/1
  Constant7/1 -> Vitis HLS2/7
  Vitis HLS2/9 -> Terminator12/1
  Constant8/1 -> Vitis HLS2/6
  Vitis HLS2/6 -> Terminator10/1
  Vitis HLS2/7 -> Terminator11/1
  Constant/1 -> Mux2/2
  rst/1 -> Register/2, Mux2/1, Scope5/1, Delay5/1
  Mux2/1 -> R_out/1, Scope6/1
  Vitis HLS2/8 -> theta_out/1, Scope2/1
  Delay5/1 -> rst_out/1

== system LinearSolver_System/ArcTan2 ==
  y_in : Inport
  sel : Inport  Port=2
  rst : Inport  Port=3
  Constant1 : hdlBasic/Constant  const=0.0  gui_display_data_type=Fixed-point  arith_type=Signed (2's comp)  n_bits=16  bin_pt=13  preci_type=Single  exp_width=8  frac_width=24  explicit_period=off  period=1  XmcBlockStatus=1  maskContainerNames=tabcontainer1  block_type=constant  block_config=sysgen:Constant_config
  Constant3 : hdlBasic/Constant  const=0.0  gui_display_data_type=Fixed-point  arith_type=Signed (2's comp)  n_bits=16  bin_pt=13  preci_type=Single  exp_width=8  frac_width=24  explicit_period=off  period=1  XmcBlockStatus=1  maskContainerNames=tabcontainer1  block_type=constant  block_config=sysgen:Constant_config
  Constant4 : hdlBasic/Constant  const=1.0  gui_display_data_type=Boolean  arith_type=Boolean  n_bits=16  bin_pt=14  preci_type=Single  exp_width=8  frac_width=24  explicit_period=off  period=1  XmcBlockStatus=1  maskContainerNames=tabcontainer1  block_type=constant  block_config=sysgen:Constant_config
  Constant5 : hdlBasic/Constant  const=0  gui_display_data_type=Boolean  arith_type=Boolean  n_bits=16  bin_pt=14  preci_type=Single  exp_width=8  frac_width=24  explicit_period=off  period=1  XmcBlockStatus=1  maskContainerNames=tabcontainer1  block_type=constant  block_config=sysgen:Constant_config
  Constant6 : hdlBasic/Constant  const=1  gui_display_data_type=Boolean  arith_type=Boolean  n_bits=16  bin_pt=13  preci_type=Single  exp_width=8  frac_width=24  explicit_period=off  period=1  XmcBlockStatus=1  maskContainerNames=tabcontainer1  block_type=constant  block_config=sysgen:Constant_config
  Constant7 : hdlBasic/Constant  const=0.0  gui_display_data_type=Fixed-point  arith_type=Signed (2's comp)  n_bits=16  bin_pt=0  preci_type=Single  exp_width=8  frac_width=24  explicit_period=off  period=1  XmcBlockStatus=1  maskContainerNames=tabcontainer1  block_type=constant  block_config=sysgen:Constant_config
  Constant8 : hdlBasic/Constant  const=0.0  gui_display_data_type=Fixed-point  arith_type=Signed (2's comp)  n_bits=16  bin_pt=13  preci_type=Single  exp_width=8  frac_width=24  explicit_period=off  period=1  XmcBlockStatus=1  maskContainerNames=tabcontainer1  block_type=constant  block_config=sysgen:Constant_config
  Delay : hdlBasic/Delay  rst=off  en=off  latency=43  reg_retiming=off  XmcBlockStatus=1  maskContainerNames=group1  block_type=delay  block_config=sysgen:Delay_config
  Mux : hdlBasic/Mux  inputs=2  en=off  latency=0  precision=Full  arith_type=Unsigned  n_bits=16  bin_pt=14  quantization=Truncate  overflow=Wrap  XmcBlockStatus=1  maskContainerNames=tabcontainer1  block_type=mux  block_config=sysgen:Mux_config
  Mux2 : hdlBasic/Mux  inputs=2  en=off  latency=0  precision=Full  arith_type=Unsigned  n_bits=16  bin_pt=14  quantization=Truncate  overflow=Wrap  XmcBlockStatus=1  maskContainerNames=tabcontainer1  block_type=mux  block_config=sysgen:Mux_config
  Negate1 : hdlBasic/Negate  precision=User Defined  arith_type="Signed  (2's comp)"  n_bits=16  bin_pt=13  quantization=Truncate  overflow=Wrap  en=off  latency=0  XmcBlockStatus=1  maskContainerNames=tabcontainer1  block_type=negate  block_config=sysgen:Negate_config
  Register : hdlBasic/Register  init=0  rst=on  en=off  XmcBlockStatus=1  maskContainerNames=tabcontainer1  block_type=register  block_config=sysgen:Register_config
  Scope : Scope
  Scope6 : Scope
  Terminator{1..7} (7 alike) : Terminator
  Vitis HLS2 : hdlBasic/Vitis HLS  anytable='..\Vitis_HLS\project6_final_hls_mc\solution1_without_back_substitution'  fast_sim=off  display_datatype=off  rate_propagation_method=Simulink system period  model_file_path=''  latency=1  block_type=vitis_hls
      settings: infoedit=This block allows including C,C++ and SystemC source files in System Generator for DSP designs.
  theta_out : Outport
  x_out : Outport  Port=2
  ready : Outport  Port=3
  R_out : Outport  Port=4
  wires:
  Constant3/1 -> Mux/2
  Mux/1 -> Mux2/3, Register/1
  Vitis HLS2/4 -> Negate1/1, x_out/1, Mux/3
  y_in/1 -> Vitis HLS2/5
  sel/1 -> Delay/1
  Delay/1 -> ready/1, Mux/1
  Vitis HLS2/5 -> Terminator3/1
  rst/1 -> Mux2/1, Register/2
  Register/1 -> Vitis HLS2/4
  Constant6/1 -> Vitis HLS2/3
  Constant7/1 -> Vitis HLS2/7
  Constant4/1 -> Vitis HLS2/2
  Constant8/1 -> Vitis HLS2/6
  Constant5/1 -> Vitis HLS2/1
  Vitis HLS2/9 -> Terminator5/1
  Vitis HLS2/6 -> Terminator4/1
  Vitis HLS2/3 -> Terminator6/1
  Vitis HLS2/2 -> Terminator1/1
  Vitis HLS2/1 -> Terminator2/1
  Vitis HLS2/7 -> Terminator7/1
  Negate1/1 -> Scope/1
  Mux2/1 -> R_out/1, Scope6/1
  Constant1/1 -> Mux2/2
  Vitis HLS2/8 -> theta_out/1

== system LinearSolver_System/ArcTan3 ==
  y_in : Inport
  sel : Inport  Port=2
  rst : Inport  Port=3
  Constant1 : hdlBasic/Constant  const=0.0  gui_display_data_type=Fixed-point  arith_type=Signed (2's comp)  n_bits=16  bin_pt=13  preci_type=Single  exp_width=8  frac_width=24  explicit_period=off  period=1  XmcBlockStatus=1  maskContainerNames=tabcontainer1  block_type=constant  block_config=sysgen:Constant_config
  Constant3 : hdlBasic/Constant  const=0.0  gui_display_data_type=Fixed-point  arith_type=Signed (2's comp)  n_bits=16  bin_pt=13  preci_type=Single  exp_width=8  frac_width=24  explicit_period=off  period=1  XmcBlockStatus=1  maskContainerNames=tabcontainer1  block_type=constant  block_config=sysgen:Constant_config
  Constant4 : hdlBasic/Constant  const=1.0  gui_display_data_type=Boolean  arith_type=Boolean  n_bits=16  bin_pt=14  preci_type=Single  exp_width=8  frac_width=24  explicit_period=off  period=1  XmcBlockStatus=1  maskContainerNames=tabcontainer1  block_type=constant  block_config=sysgen:Constant_config
  Constant5 : hdlBasic/Constant  const=0  gui_display_data_type=Boolean  arith_type=Boolean  n_bits=16  bin_pt=14  preci_type=Single  exp_width=8  frac_width=24  explicit_period=off  period=1  XmcBlockStatus=1  maskContainerNames=tabcontainer1  block_type=constant  block_config=sysgen:Constant_config
  Constant6 : hdlBasic/Constant  const=1  gui_display_data_type=Boolean  arith_type=Boolean  n_bits=16  bin_pt=13  preci_type=Single  exp_width=8  frac_width=24  explicit_period=off  period=1  XmcBlockStatus=1  maskContainerNames=tabcontainer1  block_type=constant  block_config=sysgen:Constant_config
  Constant7 : hdlBasic/Constant  const=0.0  gui_display_data_type=Fixed-point  arith_type=Signed (2's comp)  n_bits=16  bin_pt=0  preci_type=Single  exp_width=8  frac_width=24  explicit_period=off  period=1  XmcBlockStatus=1  maskContainerNames=tabcontainer1  block_type=constant  block_config=sysgen:Constant_config
  Constant8 : hdlBasic/Constant  const=0.0  gui_display_data_type=Fixed-point  arith_type=Signed (2's comp)  n_bits=16  bin_pt=13  preci_type=Single  exp_width=8  frac_width=24  explicit_period=off  period=1  XmcBlockStatus=1  maskContainerNames=tabcontainer1  block_type=constant  block_config=sysgen:Constant_config
  Delay : hdlBasic/Delay  rst=off  en=off  latency=43  reg_retiming=off  XmcBlockStatus=1  maskContainerNames=group1  block_type=delay  block_config=sysgen:Delay_config
  Mux : hdlBasic/Mux  inputs=2  en=off  latency=0  precision=Full  arith_type=Unsigned  n_bits=16  bin_pt=14  quantization=Truncate  overflow=Wrap  XmcBlockStatus=1  maskContainerNames=tabcontainer1  block_type=mux  block_config=sysgen:Mux_config
  Mux2 : hdlBasic/Mux  inputs=2  en=off  latency=0  precision=Full  arith_type=Unsigned  n_bits=16  bin_pt=14  quantization=Truncate  overflow=Wrap  XmcBlockStatus=1  maskContainerNames=tabcontainer1  block_type=mux  block_config=sysgen:Mux_config
  Register : hdlBasic/Register  init=0  rst=on  en=off  XmcBlockStatus=1  maskContainerNames=tabcontainer1  block_type=register  block_config=sysgen:Register_config
  Scope : Scope
  Scope1 : Scope
  Scope6 : Scope
  Terminator{1..7} (7 alike) : Terminator
  Vitis HLS2 : hdlBasic/Vitis HLS  anytable='..\Vitis_HLS\project6_final_hls_mc\solution1_without_back_substitution'  fast_sim=off  display_datatype=off  rate_propagation_method=Simulink system period  model_file_path=''  latency=1  block_type=vitis_hls
      settings: infoedit=This block allows including C,C++ and SystemC source files in System Generator for DSP designs.
  theta_out : Outport
  x_out : Outport  Port=2
  ready : Outport  Port=3
  R_out : Outport  Port=4
  wires:
  Constant3/1 -> Mux/2
  Vitis HLS2/4 -> x_out/1, Mux/3
  y_in/1 -> Vitis HLS2/5
  sel/1 -> Delay/1
  Delay/1 -> ready/1, Mux/1
  rst/1 -> Mux2/1, Register/2
  Mux/1 -> Mux2/3, Scope/1, Register/1
  Constant6/1 -> Vitis HLS2/3
  Constant7/1 -> Vitis HLS2/7
  Constant4/1 -> Vitis HLS2/2
  Constant8/1 -> Vitis HLS2/6
  Constant5/1 -> Vitis HLS2/1
  Register/1 -> Vitis HLS2/4, Scope1/1
  Vitis HLS2/7 -> Terminator5/1
  Vitis HLS2/9 -> Terminator6/1
  Vitis HLS2/5 -> Terminator2/1
  Vitis HLS2/6 -> Terminator7/1
  Vitis HLS2/3 -> Terminator1/1
  Vitis HLS2/2 -> Terminator3/1
  Vitis HLS2/1 -> Terminator4/1
  Mux2/1 -> R_out/1, Scope6/1
  Constant1/1 -> Mux2/2
  Vitis HLS2/8 -> theta_out/1

== system LinearSolver_System/Rotation1 ==
  y_in : Inport
  theta_in : Inport  Port=2
  rst : Inport  Port=3
  R_in : Inport  Port=4
  Constant3 : hdlBasic/Constant  const=0.0  gui_display_data_type=Fixed-point  arith_type=Signed (2's comp)  n_bits=16  bin_pt=13  preci_type=Single  exp_width=8  frac_width=24  explicit_period=off  period=1  XmcBlockStatus=1  maskContainerNames=tabcontainer1  block_type=constant  block_config=sysgen:Constant_config
  Constant4 : hdlBasic/Constant  const=1.0  gui_display_data_type=Boolean  arith_type=Boolean  n_bits=16  bin_pt=14  preci_type=Single  exp_width=8  frac_width=24  explicit_period=off  period=1  XmcBlockStatus=1  maskContainerNames=tabcontainer1  block_type=constant  block_config=sysgen:Constant_config
  Constant5 : hdlBasic/Constant  const=0  gui_display_data_type=Boolean  arith_type=Boolean  n_bits=16  bin_pt=14  preci_type=Single  exp_width=8  frac_width=24  explicit_period=off  period=1  XmcBlockStatus=1  maskContainerNames=tabcontainer1  block_type=constant  block_config=sysgen:Constant_config
  Constant6 : hdlBasic/Constant  const=0  gui_display_data_type=Boolean  arith_type=Boolean  n_bits=16  bin_pt=13  preci_type=Single  exp_width=8  frac_width=24  explicit_period=off  period=1  XmcBlockStatus=1  maskContainerNames=tabcontainer1  block_type=constant  block_config=sysgen:Constant_config
  Constant7 : hdlBasic/Constant  const=0.0  gui_display_data_type=Fixed-point  arith_type=Signed (2's comp)  n_bits=16  bin_pt=0  preci_type=Single  exp_width=8  frac_width=24  explicit_period=off  period=1  XmcBlockStatus=1  maskContainerNames=tabcontainer1  block_type=constant  block_config=sysgen:Constant_config
  Delay1 : hdlBasic/Delay  rst=off  en=off  latency=42  reg_retiming=off  XmcBlockStatus=1  maskContainerNames=group1  block_type=delay  block_config=sysgen:Delay_config
  Delay5 : hdlBasic/Delay  rst=off  en=off  latency=0  reg_retiming=off  XmcBlockStatus=1  maskContainerNames=group1  block_type=delay  block_config=sysgen:Delay_config
  Mux : hdlBasic/Mux  inputs=2  en=off  latency=0  precision=Full  arith_type=Unsigned  n_bits=16  bin_pt=14  quantization=Truncate  overflow=Wrap  XmcBlockStatus=1  maskContainerNames=tabcontainer1  block_type=mux  block_config=sysgen:Mux_config
  Mux2 : hdlBasic/Mux  inputs=2  en=off  latency=0  precision=Full  arith_type=Unsigned  n_bits=16  bin_pt=14  quantization=Truncate  overflow=Wrap  XmcBlockStatus=1  maskContainerNames=tabcontainer1  block_type=mux  block_config=sysgen:Mux_config
  Register : hdlBasic/Register  init=0  rst=on  en=off  XmcBlockStatus=1  maskContainerNames=tabcontainer1  block_type=register  block_config=sysgen:Register_config
  Scope{,1..2,6} (4 alike) : Scope
  Terminator{1..6} (6 alike) : Terminator
  Vitis HLS2 : hdlBasic/Vitis HLS  anytable='..\Vitis_HLS\project6_final_hls_mc\solution1_without_back_substitution'  fast_sim=off  display_datatype=off  rate_propagation_method=Simulink system period  model_file_path=''  latency=1  block_type=vitis_hls
      settings: infoedit=This block allows including C,C++ and SystemC source files in System Generator for DSP designs.
  theta_out : Outport
  y_out : Outport  Port=2
  x_out : Outport  Port=3
  R_out : Outport  Port=4
  rst_out : Outport  Port=5
  wires:
  Mux/1 -> Mux2/3, Scope/1, Register/1
  Vitis HLS2/4 -> Scope2/1, x_out/1, Mux/3
  y_in/1 -> Vitis HLS2/5
  Constant3/1 -> Mux/2
  Vitis HLS2/5 -> Mux/1
  Vitis HLS2/6 -> y_out/1
  Register/1 -> Vitis HLS2/4
  rst/1 -> Delay1/1, Scope1/1, Register/2, Mux2/1
  Constant5/1 -> Vitis HLS2/1
  Constant4/1 -> Vitis HLS2/2
  Constant7/1 -> Vitis HLS2/7
  Constant6/1 -> Vitis HLS2/3
  Vitis HLS2/8 -> Terminator3/1
  Vitis HLS2/9 -> Terminator1/1
  Vitis HLS2/2 -> Terminator4/1
  Vitis HLS2/1 -> Terminator5/1
  Vitis HLS2/3 -> Terminator2/1
  Vitis HLS2/7 -> Terminator6/1
  Mux2/1 -> R_out/1, Scope6/1
  R_in/1 -> Mux2/2
  Delay5/1 -> Vitis HLS2/6, theta_out/1
  theta_in/1 -> Delay5/1
  Delay1/1 -> rst_out/1
